simulink model "dynsim_test_urdf_complesso"  (R2020a)
settings: Solver=FixedStepAuto  StartTime=0.0  StopTime=15  FixedStep=0.001  RelTol=1e-3
libraries: robotmaniplib x1, simulink x1
settings Model: SimulationMode=accelerator  Creator=bascetta  LastModifiedBy=alberto
settings OptimizationCC: EnhancedBackFolding=on  PassReuseOutputArgsAs=Individual arguments  ZeroExternalMemoryAtStartup=off  ZeroInternalMemoryAtStartup=off  MaxStackSize=64  OptimizeBlockOrder=speed  DifferentSizesBufferReuse=on  OptimizationCustomize=off  EfficientTunableParamExpr=on
settings DebuggingCC: ParameterTunabilityLossMsg=error
settings HardwareCC: ProdBitPerPointer=32  ProdBitPerSizeT=32  ProdBitPerPtrDiffT=32  ProdLargestAtomicFloat=None  ProdIntDivRoundTo=Undefined  ProdEndianess=Unspecified  ProdWordSize=32  ProdHWDeviceType=Generic->Unspecified (assume 32-bit Generic)
settings RTWCC: SystemTargetFile=ert.tlc  HardwareBoard=Robot Operating System (ROS)  TemplateMakefile=ert_default_tmf  GenerateReport=on  Toolchain=Catkin  IncludeHyperlinkInReport=on  LaunchReport=on  TargetLang=C++  GenerateTraceInfo=on  GenerateTraceReport=on  GenerateTraceReportSl=on  GenerateTraceReportSf=on  GenerateTraceReportEml=on
settings CodeAppCC: ForceParamTrailComments=on  IgnoreCustomStorageClasses=off  OperatorAnnotations=on  SimulinkDataObjDesc=on  SFDataObjDesc=on  InsertBlockDesc=on
settings ERTTargetCC: SupportContinuousTime=on  SupportVariableSizeSignals=on

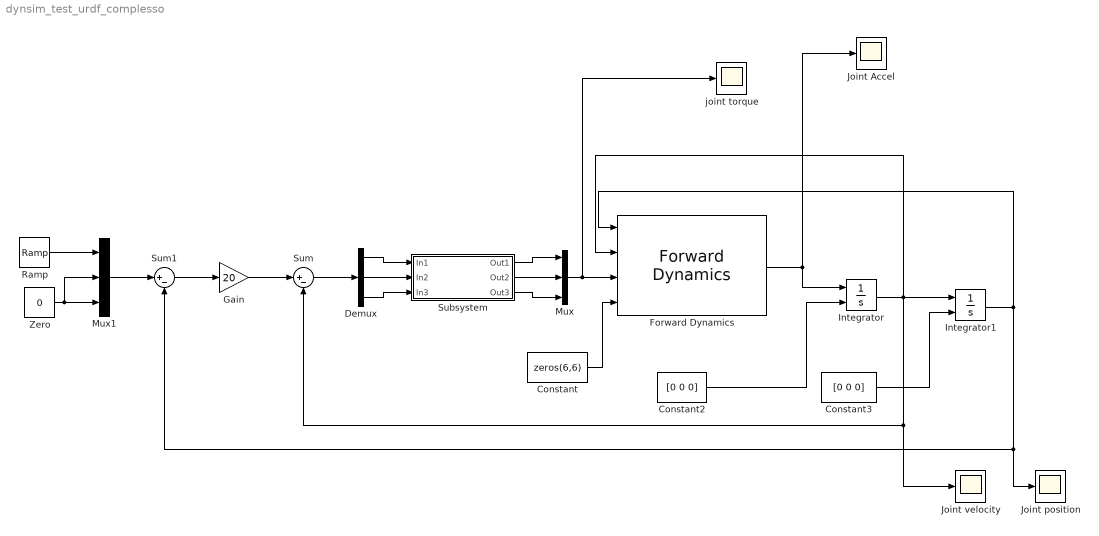
== system dynsim_test_urdf_complesso ==
  Constant : Constant  Value=zeros(6,6)
  Constant2 : Constant  Value=[0 0 0]
  Constant3 : Constant  Value=[0 0 0]
  Demux : Demux  Outputs=3
  Forward Dynamics : robotmaniplib/Forward Dynamics  RigidBodyTree=robot_edo_nuove_inerzie  SimulateUsing=Interpreted execution
  Gain : Gain  Gain=20
  Integrator : Integrator  InitialConditionSource=external
  Integrator1 : Integrator  InitialConditionSource=external
  Joint Accel : Scope
  Joint position : Scope
  Joint velocity : Scope
  Mux : Mux  Inputs=3
  Mux1 : Mux  Inputs=3
  Ramp : simulink/Sources/Ramp  slope=1  start=0  InitialOutput=0
  Subsystem : Subsystem
  Sum : Sum  Inputs=|+-
  Sum1 : Sum  Inputs=|+-
  Zero : Constant  Value=0  OutDataTypeStr=Inherit: Inherit via back propagation
  joint torque : Scope
  wires:
  Constant/1 -> Forward Dynamics/4
  Forward Dynamics/1 -> Integrator/1, Joint Accel/1
  Integrator1/1 -> Forward Dynamics/1, Sum1/2, Joint position/1
  Constant2/1 -> Integrator/2
  Constant3/1 -> Integrator1/2
  Integrator/1 -> Sum/2, Joint velocity/1, Forward Dynamics/2, Integrator1/1
  Sum/1 -> Demux/1
  Demux/1 -> Subsystem/1(In1)
  Demux/2 -> Subsystem/2(In2)
  Demux/3 -> Subsystem/3(In3)
  Subsystem/1(Out1) -> Mux/1
  Subsystem/2(Out2) -> Mux/2
  Subsystem/3(Out3) -> Mux/3
  Mux/1 -> joint torque/1, Forward Dynamics/3
  Gain/1 -> Sum/1
  Sum1/1 -> Gain/1
  Mux1/1 -> Sum1/1
  Ramp/1 -> Mux1/1
  Zero/1 -> Mux1/2, Mux1/3

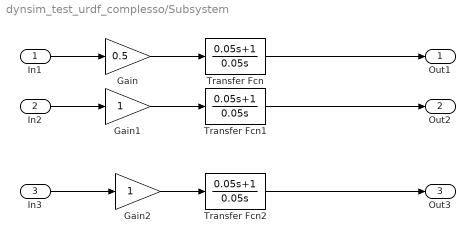
== system dynsim_test_urdf_complesso/Subsystem ==
  In1 : Inport
  In2 : Inport  Port=2
  In3 : Inport  Port=3
  Gain : Gain  Gain=0.5
  Gain1 : Gain
  Gain2 : Gain
  Transfer Fcn : TransferFcn  Numerator=[0.05 1]  Denominator=[0.05 0]
  Transfer Fcn1 : TransferFcn  Numerator=[0.05 1]  Denominator=[0.05 0]
  Transfer Fcn2 : TransferFcn  Numerator=[0.05 1]  Denominator=[0.05 0]
  Out1 : Outport
  Out2 : Outport  Port=2
  Out3 : Outport  Port=3
  wires:
  Transfer Fcn/1 -> Out1/1
  In1/1 -> Gain/1
  Gain/1 -> Transfer Fcn/1
  Transfer Fcn2/1 -> Out3/1
  Transfer Fcn1/1 -> Out2/1
  In2/1 -> Gain1/1
  Gain1/1 -> Transfer Fcn1/1
  Gain2/1 -> Transfer Fcn2/1
  In3/1 -> Gain2/1
